simulink model "driver_model_b_upd (2)"  (R2023a)
settings: Solver=FixedStepDiscrete  StartTime=0  StopTime=700  FixedStep=0.0005  RelTol=1e-3  AbsTol=1e-6
InitFcn:
  | R2D = 180/pi;
undefined symbols (not defined in the file or in its folder): b_hat_Max, SrsLrn_BrkPedDownLim, SrsLrn_BrkPedUpLim, SrsLrn_EKF_Q1, SrsLrn_EKF_Q2, SrsLrn_ExitAccPedLim, SrsLrn_Lamda1, SrsLrn_Lamda2, SrsLrn_LongAccDownLim, SrsLrn_LongAccUpLim, SrsLrn_State1Cnt, SrsLrn_State2Cnt, SrsLrn_State5Cnt, SrsLrn_State6Cnt, SrsLrn_State7Cnt, SrsLrn_UpdBrkPedDown, SrsLrn_UpdBrkPedUp, tau_hat_Max
libraries: simulink x11, slpidlib x2, Solver_SF x1
(part 1 of 2)
settings Model: ExtModeTrigMode=oneshot  Creator=jhu  LastModifiedBy=SM-PC
settings SolverCC: AutoScaleAbsTol=off  AlgebraicLoopSolver=TrustRegion
settings DataIOCC: SaveFormat=Array  ReturnWorkspaceOutputs=off  SignalLoggingName=sigsOut
settings OptimizationCC: BlockReduction=off  BooleanDataType=off  ExpressionDepthLimit=2147483647  InitFltsAndDblsToZero=on  LifeSpan=inf
settings DebuggingCC: SaveWithParameterizedLinksMsg=none  UnderspecifiedInitializationDetection=Classic  MergeDetectMultiDrivingBlocksExec=none  SignalResolutionControl=TryResolveAllWithWarning  MultiTaskDSMMsg=warning  MultiTaskCondExecSysMsg=none  ParameterPrecisionLossMsg=none  FcnCallInpInsideContextMsg=warning  UnconnectedInputMsg=warning  UnconnectedOutputMsg=warning  UnconnectedLineMsg=warning  StateNameClashWarn=warning  SFUnexpectedBacktrackingDiag=warning  SFNoUnconditionalDefaultTransitionDiag=warning  ArithmeticOperatorsInVariantConditions=warning
settings HardwareCC: ProdBitPerPointer=32  ProdBitPerSizeT=32  ProdBitPerPtrDiffT=32  ProdLargestAtomicFloat=None  ProdIntDivRoundTo=Undefined  ProdEndianess=Unspecified  ProdWordSize=32  ProdHWDeviceType=32-bit Generic  TargetHWDeviceType=32-bit Generic  TargetUnknown=on  ProdEqTarget=off
settings ModelReferenceCC: ModelReferenceMinAlgLoopOccurrences=on  PropagateSignalLabelsOutOfModel=off
settings SFSimCC: SimUseLocalCustomCode=off  CustomCodeUndefinedFunction=UseInterfaceOnly
settings RTWCC: TemplateMakefile=grt_vc.tmf  RTWUseLocalCustomCode=off
settings CodeAppCC: StateflowObjectComments=on
settings GRTTargetCC: TargetFcnLib=ansi_tfl_tmw.mat  TargetLangStandard=C89/C90 (ANSI)  CombineOutputUpdateFcns=off  GRTInterface=on
settings ConfigComp: CovMetricSettings=dw  CovSaveCumulativeToWorkspaceVar=on  CovSaveSingleToWorkspaceVar=on  CovExternalEMLEnable=off

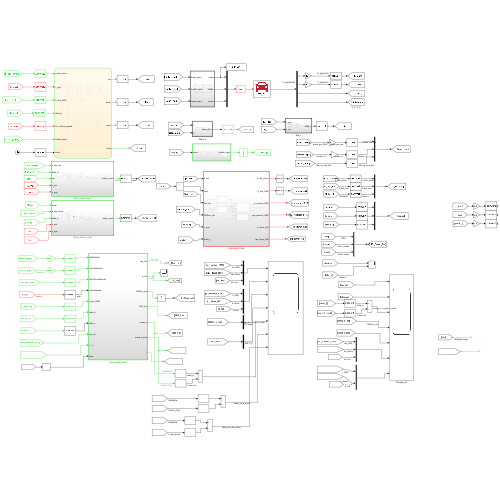
[thumbnail: Simulink's stored preview of the top-level diagram]
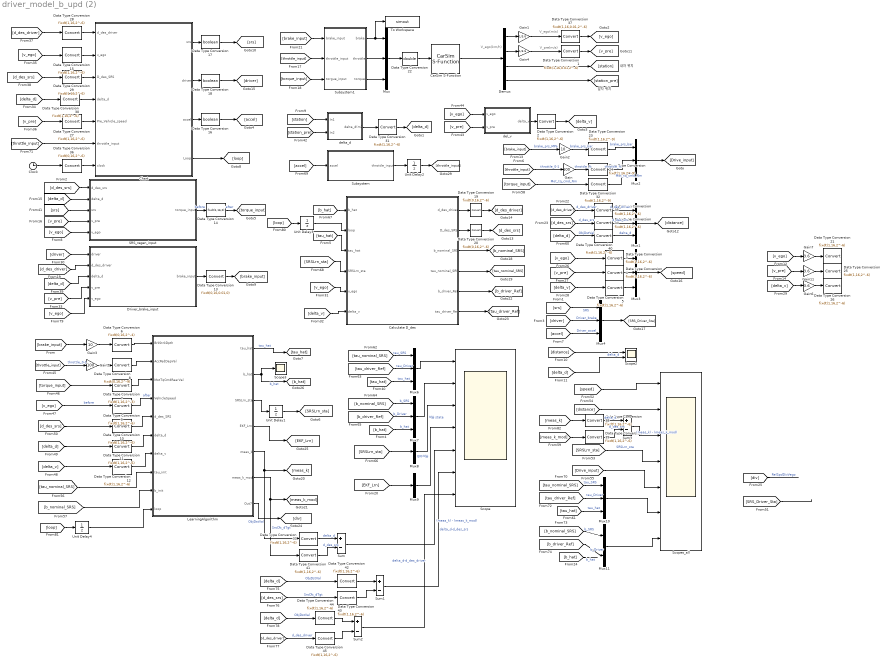
== system driver_model_b_upd (2) ==
  note: V_ego(m/s)
  note: V_pre(m/s)
  note: V_ego(km/h)
  Calculate D_des : Subsystem  TreatAsAtomicUnit=on  SystemSampleTime=0.01
      settings: MinAlgLoopOccurrences=on
  CarSim S-Function : Solver_SF/CarSim S-Function  Priority=1  SIMFILE=simfile.sim  Run_RTs=off  vs_state_ind=Run  StopMode_ind=Vehicle Model
  Chart : Stateflow chart  TreatAsAtomicUnit=on  SystemSampleTime=0.01
  Clock : Clock
  Data Type Conversion1 : DataTypeConversion  OutMin=[0]  OutMax=[300]  OutDataTypeStr=fixdt(1,16,0.01,2^-6)  RndMeth=Simplest  SaturateOnIntegerOverflow=off
  Data Type Conversion{10,29,33..35,38..45} (13 alike) : DataTypeConversion  OutDataTypeStr=fixdt(1,16,2^-6)  SaturateOnIntegerOverflow=off  RndMeth=Floor
  Data Type Conversion{2..5,9,11..12,15,21,25..27,31} (13 alike) : DataTypeConversion  OutDataTypeStr=fixdt(1,16,2^-6)  RndMeth=Simplest  SaturateOnIntegerOverflow=off
  Data Type Conversion13 : DataTypeConversion  OutDataTypeStr=fixdt(0,16,0.01,0)  SaturateOnIntegerOverflow=off  RndMeth=Floor
  Data Type Conversion14 : DataTypeConversion  OutDataTypeStr=fixdt(1,16,0)  RndMeth=Nearest  SaturateOnIntegerOverflow=off
  Data Type Conversion16 : DataTypeConversion  OutDataTypeStr=boolean  SaturateOnIntegerOverflow=off  RndMeth=Floor
  Data Type Conversion17 : DataTypeConversion  OutDataTypeStr=boolean  SaturateOnIntegerOverflow=off  RndMeth=Floor
  Data Type Conversion18 : DataTypeConversion  OutDataTypeStr=boolean  SaturateOnIntegerOverflow=off  RndMeth=Floor
  Data Type Conversion19 : DataTypeConversion  OutDataTypeStr=fixdt(0,16,2^-6)  SaturateOnIntegerOverflow=off  RndMeth=Floor
  Data Type Conversion20 : DataTypeConversion  OutDataTypeStr=fixdt(0,16,2^-6)  SaturateOnIntegerOverflow=off  RndMeth=Floor
  Data Type Conversion22 : DataTypeConversion  OutDataTypeStr=double  SaturateOnIntegerOverflow=off  RndMeth=Floor
  Data Type Conversion23 : DataTypeConversion  OutDataTypeStr=fixdt(1,16,2^-9)  SaturateOnIntegerOverflow=off  RndMeth=Floor
  Data Type Conversion24 : DataTypeConversion  OutDataTypeStr=fixdt(1,16,2^-9)  SaturateOnIntegerOverflow=off  RndMeth=Floor
  Data Type Conversion28 : DataTypeConversion  OutDataTypeStr=fixdt(1,16,2^-6)  RndMeth=Nearest  SaturateOnIntegerOverflow=off
  Data Type Conversion30 : DataTypeConversion  OutDataTypeStr=fixdt(1,16,2^-6)  RndMeth=Nearest  SaturateOnIntegerOverflow=off
  Data Type Conversion32 : DataTypeConversion  OutDataTypeStr=fixdt(1,16,2^-9)  SaturateOnIntegerOverflow=off  RndMeth=Floor
  Data Type Conversion36 : DataTypeConversion  OutDataTypeStr=fixdt(0,16,2^-6)  SaturateOnIntegerOverflow=off  RndMeth=Floor
  Data Type Conversion37 : DataTypeConversion  OutDataTypeStr=fixdt(1,16,0.01,2^-6)  RndMeth=Simplest  SaturateOnIntegerOverflow=off
  Data Type Conversion6 : DataTypeConversion  OutDataTypeStr=fixdt(0,16,2^-4)  SaturateOnIntegerOverflow=off  RndMeth=Floor
  Data Type Conversion7 : DataTypeConversion  OutDataTypeStr=fixdt(1,16,2^-3)  SaturateOnIntegerOverflow=off  RndMeth=Floor
  Data Type Conversion8 : DataTypeConversion  OutDataTypeStr=fixdt(0,16,2^-9)  SaturateOnIntegerOverflow=off  RndMeth=Floor
  Demux : Demux
  Driver_brake_input : Subsystem  TreatAsAtomicUnit=on  SystemSampleTime=0.01
  Gain : Gain  Gain=100
  Gain1 : Gain  Gain=1/3.6
  Gain11 : Gain  Gain=3.6
  Gain2 : Gain  Gain=10
  Gain3 : Gain  Gain=10
  Gain4 : Gain  Gain=1/3.6
  Gain5 : Gain  Gain=100
  Gain6 : Gain  Gain=3.6
  Gain7 : Gain  Gain=3.6
  LearningAlgorithm : Subsystem  TreatAsAtomicUnit=on  SystemSampleTime=0.01
  Mux{,1..4,6..7,10} (8 alike) : Mux  Inputs=3
  Mux11 : Mux  Inputs=2
  Mux8 : Mux  Inputs=1
  Mux9 : Mux  Inputs=1
  SRS_regen_input : Subsystem  TreatAsAtomicUnit=on  SystemSampleTime=0.01
  Scope : Scope  NumInputPorts=7
  Scope2 : Scope  NumInputPorts=2
  Scope3 : Scope
  Scopes_all : Scope  NumInputPorts=7
  Subsystem : Subsystem  TreatAsAtomicUnit=on  SystemSampleTime=0.01
      settings: MinAlgLoopOccurrences=on
  Subsystem1 : Subsystem  TreatAsAtomicUnit=on  SystemSampleTime=0.0005
  Sum{,1..3} (4 alike) : Sum  Inputs=+-
  To Workspace : ToWorkspace  VariableName=simout  SaveFormat=Timeseries  SampleTime=-1
  Unit Delay1 : UnitDelay  SampleTime=0.01  HasFrameUpgradeWarning=on
  Unit Delay2 : UnitDelay  SampleTime=0.01  HasFrameUpgradeWarning=on
  Unit Delay3 : UnitDelay  InitialCondition=1  SampleTime=0.01  HasFrameUpgradeWarning=on
  Unit Delay4 : UnitDelay  InitialCondition=1  SampleTime=0.01  HasFrameUpgradeWarning=on
  del_v : Subsystem  TreatAsAtomicUnit=on  SystemSampleTime=0.01
  delta_d : Subsystem  TreatAsAtomicUnit=on  SystemSampleTime=0.01
  wires:
  Gain1/1 -> Data Type Conversion37/1
  Mux1/1 -> [distance]
  Mux2/1 -> [Drive_input]
  [brake_input] -> Gain2/1  "brake_prs_MPa"
  [d_des_driver] -> Data Type Conversion35/1  "d_des_driver"
  [d_des_srs] -> Data Type Conversion34/1  "d_des_srs"
  [delta_d] -> Data Type Conversion30/1
  [v_pre] -> Data Type Conversion27/1
  [d_des_driver] -> Data Type Conversion28/1
  [d_des_srs] -> Data Type Conversion29/1
  Chart/1(srs) -> Data Type Conversion17/1
  Chart/2(driver) -> Data Type Conversion18/1
  [driver] -> Mux4/2  "Driver_brake"
  [srs] -> Mux4/1  "SRS"
  Mux4/1 -> [SRS_Driver_Sta]
  Chart/3(accel) -> Data Type Conversion16/1
  [throttle_input] -> Gain/1  "throttle_0-1"
  [accel] -> Mux4/3  "Driver_accel"
  Mux3/1 -> [speed]
  [d_des_driver] -> Driver_brake_input/2(d_des_driver)
  [delta_d] -> Driver_brake_input/3(delta_d)
  Driver_brake_input/1(brake_input) -> Data Type Conversion13/1
  [d_des_srs] -> SRS_regen_input/1(d_des_srs)
  [delta_d] -> SRS_regen_input/2(delta_d)
  [driver] -> Driver_brake_input/1(driver)
  [srs] -> SRS_regen_input/3(srs)
  SRS_regen_input/1(torque_input) -> Data Type Conversion14/1  "before"
  [v_pre] -> SRS_regen_input/4(v_pre)
  [v_pre] -> Driver_brake_input/4(v_pre)
  Gain4/1 -> Data Type Conversion1/1
  Demux/2 -> Gain4/1
  Gain/1 -> Data Type Conversion24/1  "throttle_%"
  Gain2/1 -> Data Type Conversion23/1  "brake_prs_bar"
  [brake_input] -> Gain3/1
  Gain3/1 -> Data Type Conversion6/1
  [throttle_input] -> Gain5/1  "throttle_0-1"
  Gain5/1 -> Data Type Conversion8/1
  [torque_input] -> Data Type Conversion7/1
  [v_ego] -> Data Type Conversion9/1  "before"
  [delta_d] -> Data Type Conversion11/1
  [d_des_srs] -> Data Type Conversion10/1
  [v_ego] -> Data Type Conversion3/1
  [v_pre] -> Data Type Conversion4/1
  [delta_v] -> Data Type Conversion5/1
  [SRS_Driver_Sta] -> ?
  [SRSLrn_sta] -> Scopes_all/4  "SRSLrn_sta"
  [speed] -> Scopes_all/1
  [distance] -> Scopes_all/2
  [Drive_input] -> Scopes_all/5
  [tau_nominal_SRS] -> LearningAlgorithm/8(tau_init)
  LearningAlgorithm/1(tau_hat) -> [tau_hat]  "tau_hat"
  LearningAlgorithm/2(b_hat) -> [b_hat], Scope3/1  "b_hat"
  Mux6/1 -> Scope/1
  Mux7/1 -> Scope/2
  [tau_nominal_SRS] -> Mux6/1  "tau_SRS"
  [tau_driver_Ref] -> Mux6/2  "tau_Driver"
  [b_nominal_SRS] -> Mux7/1  "b_SRS"
  [b_driver_Ref] -> Mux7/2  "b_Driver"
  Clock/1 -> Data Type Conversion36/1
  [b_nominal_SRS] -> LearningAlgorithm/9(b_init)
  LearningAlgorithm/3(SRSLrn_sta) -> Unit Delay1/1
  Unit Delay1/1 -> [SRSLrn_sta]
  LearningAlgorithm/4(EKF_Lrn) -> [EKF_Lrn]
  [EKF_Lrn] -> Mux9/1
  [SRSLrn_sta] -> Mux8/1
  Mux8/1 -> Scope/3  "학습 state"
  Mux9/1 -> Scope/4  "EKF학습"
  [b_hat] -> Mux7/3  "b_hat"
  [tau_hat] -> Mux6/3  "tau_hat"
  [accel] -> Subsystem/1(accel)
  Calculate D_des/3(b_nominal_SRS) -> [b_nominal_SRS]
  [tau_hat] -> Calculate D_des/3(tau_hat)
  Calculate D_des/6(tau_driver_Ref) -> [tau_driver_Ref]
  Calculate D_des/4(tau_nominal_SRS) -> [tau_nominal_SRS]
  Calculate D_des/1(d_des_driver) -> Data Type Conversion19/1
  Calculate D_des/5(b_driver_Ref) -> [b_driver_Ref]
  [SRSLrn_sta] -> Calculate D_des/4(SRSLrn_sta)
  Calculate D_des/2(D_des_SRS) -> Data Type Conversion20/1
  [v_ego] -> Calculate D_des/5(v_ego)
  [delta_v] -> Calculate D_des/6(delta_v)
  [b_hat] -> Calculate D_des/1(b_hat)
  CarSim S-Function/1 -> Demux/1
  Data Type Conversion37/1 -> [v_ego]
  Data Type Conversion1/1 -> [v_pre]
  Data Type Conversion2/1 -> [delta_v]
  Data Type Conversion3/1 -> Mux3/1
  Data Type Conversion4/1 -> Mux3/2
  Data Type Conversion5/1 -> Mux3/3
  Data Type Conversion6/1 -> LearningAlgorithm/1(BrkStrkDpth)
  Data Type Conversion8/1 -> LearningAlgorithm/2(AccPedDepVal)
  Data Type Conversion7/1 -> LearningAlgorithm/3(MotTqCmdRearVal)
  Data Type Conversion9/1 -> LearningAlgorithm/4(VehicleSpeed)  "after"
  Data Type Conversion10/1 -> LearningAlgorithm/5(d_des_SRS)
  Data Type Conversion11/1 -> LearningAlgorithm/6(delta_d)
  Data Type Conversion12/1 -> LearningAlgorithm/7(delta_v)
  Mux/1 -> Data Type Conversion22/1
  Data Type Conversion14/1 -> [torque_input]  "after"
  Data Type Conversion16/1 -> [accel]
  Data Type Conversion17/1 -> [srs]
  Data Type Conversion18/1 -> [driver]
  Subsystem/1(throttle_input) -> Unit Delay2/1
  Data Type Conversion19/1 -> [d_des_driver]
  Data Type Conversion20/1 -> [d_des_srs]
  Data Type Conversion22/1 -> CarSim S-Function/1
  Data Type Conversion23/1 -> Mux2/1  "brake_prs_bar"
  Data Type Conversion24/1 -> Mux2/2  "throttle_%"
  Data Type Conversion15/1 -> Chart/2(v_ego)
  Data Type Conversion28/1 -> Chart/1(d_des_driver)
  Data Type Conversion29/1 -> Chart/3(D_des_SRS)
  Data Type Conversion30/1 -> Chart/4(delta_d)
  Data Type Conversion27/1 -> Chart/5(Pre_Vehicle_speed)
  [throttle_input] -> Chart/6(throttle_input)
  Data Type Conversion34/1 -> Mux1/2  "d_des_srs"
  Data Type Conversion35/1 -> Mux1/1  "d_des_driver"
  Data Type Conversion13/1 -> [brake_input]
  Data Type Conversion36/1 -> Chart/7(clock)
  Demux/1 -> Gain1/1
  [v_ego] -> SRS_regen_input/5(v_ego)
  [v_ego] -> Data Type Conversion15/1
  [distance] -> Scope2/1
  [delta_d] -> Scope2/2  "delta_d"
  Demux/3 -> [station]
  Demux/4 -> [station_pre]
  Data Type Conversion31/1 -> [delta_d]
  [v_ego] -> del_v/1(v_ego)
  [v_pre] -> del_v/2(v_pre)
  del_v/1(delta_v) -> Data Type Conversion2/1
  [station] -> delta_d/1(In1)
  [station_pre] -> delta_d/2(In2)
  delta_d/1(delta_d(m)) -> Data Type Conversion31/1
  [brake_input] -> Subsystem1/1(brake_input)
  [throttle_input] -> Subsystem1/2(throttle_input)
  [torque_input] -> Subsystem1/3(torgue_input)
  Subsystem1/1(brake) -> To Workspace/1, Mux/1
  Subsystem1/2(throttle) -> Mux/2
  Subsystem1/3(torque) -> Mux/3
  [delta_v] -> Data Type Conversion12/1
  Gain6/1 -> Data Type Conversion26/1
  [delta_v] -> Gain6/1
  [v_pre] -> Gain11/1
  Gain11/1 -> Data Type Conversion25/1
  [v_ego] -> Gain7/1
  Gain7/1 -> Data Type Conversion21/1
  [torque_input] -> Data Type Conversion32/1  "Mot_tq_cmd_Nm"
  Data Type Conversion32/1 -> Mux2/3  "Mot_tq_cmd_Nm"
  [delta_d] -> Data Type Conversion40/1  "ObjDstVal"
  Data Type Conversion40/1 -> Mux1/3  "delta_d"
  Mux10/1 -> Scopes_all/6
  [b_driver_Ref] -> Mux11/2  "b_Driver"
  [b_nominal_SRS] -> Mux11/1  "b_SRS"
  Mux11/1 -> Scopes_all/7
  [tau_driver_Ref] -> Mux10/2  "tau_Driver"
  [tau_nominal_SRS] -> Mux10/1  "tau_SRS"
  [tau_hat] -> Mux10/3  "tau_hat"
  [b_hat] -> ?  "b_hat"
  Sum/1 -> Scope/5  "(meas_k) - (meas_k_mod)"
  Data Type Conversion41/1 -> Sum/2  "d_des_srs"
  LearningAlgorithm/5(meas_k) -> Data Type Conversion33/1, [meas_k]  "ObjDstVal"
  Data Type Conversion33/1 -> Sum/1  "delta_d"
  LearningAlgorithm/6(meas_k_mod) -> Data Type Conversion41/1, [meas_k_mod]  "SrsCfc_dTgt"
  Data Type Conversion43/1 -> Sum1/2
  Data Type Conversion42/1 -> Sum1/1
  Sum1/1 -> Scope/6  "delta_d-d_des_srs"
  [delta_d] -> Data Type Conversion42/1  "ObjDstVal"
  [d_des_srs] -> Data Type Conversion43/1  "SrsCfc_dTgt"
  Chart/4(Loop) -> [loop]
  Data Type Conversion44/1 -> Sum2/1
  Data Type Conversion45/1 -> Sum2/2
  [delta_d] -> Data Type Conversion44/1  "ObjDstVal"
  [d_des_driver] -> Data Type Conversion45/1  "d_des_driver"
  Sum2/1 -> Scope/7  "delta_d-d_des_driver"
  [v_ego] -> Driver_brake_input/5(v_ego)
  [loop] -> Unit Delay3/1
  Unit Delay3/1 -> Calculate D_des/2(loop)
  [loop] -> Unit Delay4/1
  Unit Delay4/1 -> LearningAlgorithm/10(loop)
  Unit Delay2/1 -> [throttle_input]
  LearningAlgorithm/7(Out7) -> [div]
  [div] -> ?  "RelSpdDivVego"
  Data Type Conversion39/1 -> Sum3/2  "d_des_srs"
  Data Type Conversion38/1 -> Sum3/1  "delta_d"
  [meas_k] -> Data Type Conversion38/1
  [meas_k_mod] -> Data Type Conversion39/1
  Sum3/1 -> Scopes_all/3  "(meas_k) - (meas_k_mod)"

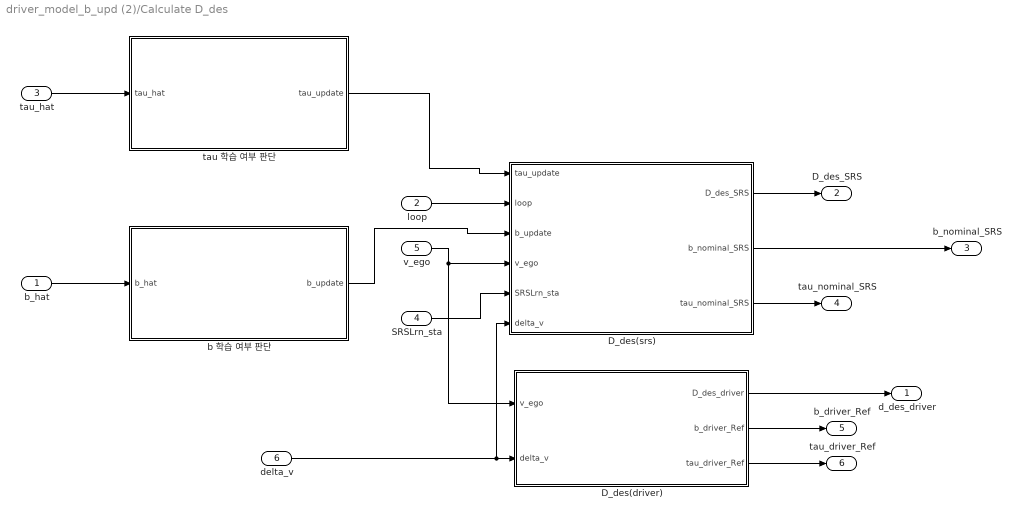
== system driver_model_b_upd (2)/Calculate D_des ==
  b_hat : Inport
  loop : Inport  Port=2
  tau_hat : Inport  Port=3
  SRSLrn_sta : Inport  Port=4
  v_ego : Inport  Port=5
  delta_v : Inport  Port=6
  D_des(driver) : Subsystem
  D_des(srs) : Subsystem
  b 학습 여부 판단 : Subsystem
  tau 학습 여부 판단 : Subsystem
  d_des_driver : Outport
  D_des_SRS : Outport  Port=2
  b_nominal_SRS : Outport  Port=3
  tau_nominal_SRS : Outport  Port=4
  b_driver_Ref : Outport  Port=5
  tau_driver_Ref : Outport  Port=6
  wires:
  v_ego/1 -> D_des(driver)/1(v_ego), D_des(srs)/4(v_ego)
  delta_v/1 -> D_des(driver)/2(delta_v), D_des(srs)/6(delta_v)
  D_des(srs)/1(D_des_SRS) -> D_des_SRS/1
  D_des(driver)/1(D_des_driver) -> d_des_driver/1
  D_des(srs)/2(b_nominal_SRS) -> b_nominal_SRS/1
  D_des(srs)/3(tau_nominal_SRS) -> tau_nominal_SRS/1
  D_des(driver)/2(b_driver_Ref) -> b_driver_Ref/1
  D_des(driver)/3(tau_driver_Ref) -> tau_driver_Ref/1
  SRSLrn_sta/1 -> D_des(srs)/5(SRSLrn_sta)
  b_hat/1 -> b 학습 여부 판단/1(b_hat)
  b 학습 여부 판단/1(b_update) -> D_des(srs)/3(b_update)
  tau_hat/1 -> tau 학습 여부 판단/1(tau_hat)
  tau 학습 여부 판단/1(tau_update) -> D_des(srs)/1(tau_update)
  loop/1 -> D_des(srs)/2(loop)

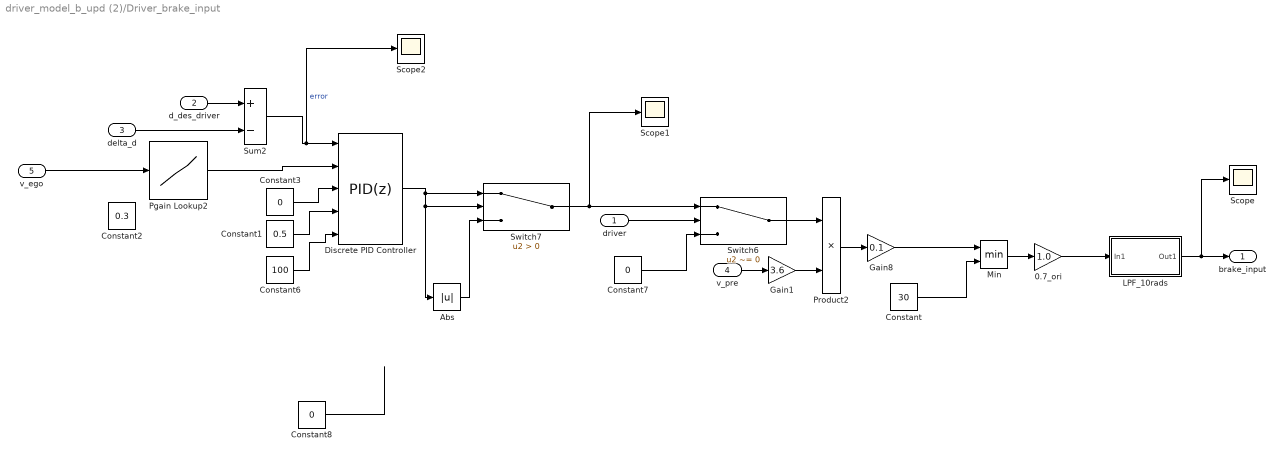
== system driver_model_b_upd (2)/Driver_brake_input ==
  driver : Inport
  d_des_driver : Inport  Port=2
  delta_d : Inport  Port=3
  v_pre : Inport  Port=4
  v_ego : Inport  Port=5
  0.7_ori : Gain  Gain=1.0
  Abs : Abs  SaturateOnIntegerOverflow=off
  Constant : Constant  Value=30
  Constant1 : Constant  Value=0.5
  Constant2 : Constant  Value=0.3
  Constant3 : Constant  Value=0
  Constant6 : Constant  Value=100
  Constant7 : Constant  Value=0
  Constant8 : Constant  Value=0
  Discrete PID Controller : slpidlib/PID Controller  Controller=PID  Form=Parallel  TimeDomain=Discrete-time  UseExternalTs=off  SampleTime=0.01  IntegratorMethod=Forward Euler  FilterMethod=Forward Euler  ControllerParametersSource=external  P=1  I=1  UseKiTs=off  D=0  N=100  UseFilter=on  TunerSelectOption=Transfer Function Based (PID Tuner App)  InitialConditionSource=internal  InitialConditionForIntegrator=0  InitialConditionForFilter=0  DifferentiatorICPrevScaledInput=0  ExternalReset=none  TrackingMode=off  Kt=1  LimitOutput=off  SatLimitsSource=internal  UpperSaturationLimit=inf  LowerSaturationLimit=-inf  LinearizeAsGain=off  AntiWindupMode=none  Kb=1  LimitIntegrator=off  UpperIntegratorSaturationLimit=inf  LowerIntegratorSaturationLimit=-inf  POutMin=[]  POutMax=[]  IOutMin=[]  IOutMax=[]  DOutMin=[]  DOutMax=[]  NOutMin=[]  NOutMax=[]  SumOutMin=[]  SumOutMax=[]  SaturationOutMin=[]  SaturationOutMax=[]  PParamMin=[]  PParamMax=[]  IParamMin=[]  IParamMax=[]  DParamMin=[]  DParamMax=[]  NParamMin=[]  NParamMax=[]  KbParamMin=[]  KbParamMax=[]  KtParamMin=[]  KtParamMax=[]  KbOutMin=[]  KbOutMax=[]  KtOutMin=[]  KtOutMax=[]  IntegratorOutMin=[]  IntegratorOutMax=[]  FilterOutMin=[]  FilterOutMax=[]  SumI1OutMin=[]  SumI1OutMax=[]  SumI2OutMin=[]  SumI2OutMax=[]  SumI3OutMin=[]  SumI3OutMax=[]  SumI4OutMin=[]  SumI4OutMax=[]  SumDOutMin=[]  SumDOutMax=[]  DifferentiatorOutMin=[]  DifferentiatorOutMax=[]  FilterDiffOutCoefMin=[]  FilterDiffOutCoefMax=[]  ReciprocalOutMin=[]  ReciprocalOutMax=[]  SumDenOutMin=[]  SumDenOutMax=[]  SumNumOutMin=[]  SumNumOutMax=[]  DivideOutMin=[]  DivideOutMax=[]  UdiffTsProdOutMin=[]  UdiffTsProdOutMax=[]  NTsProdOutMin=[]  NTsProdOutMax=[]  UintegralTsProdOutMin=[]  UintegralTsProdOutMax=[]  UngainTsProdOutMin=[]  UngainTsProdOutMax=[]  ClampingZeroOutDataTypeStr=Inherit: Inherit via back propagation  ClampingZeroOutMin=[]  ClampingZeroOutMax=[]  FilterDenConstantOutDataTypeStr=Inherit: Inherit via back propagation  FilterDenConstantOutMin=[]  FilterDenConstantOutMax=[]  PCopyOutDataTypeStr=Inherit: Inherit via back propagation  PCopyOutMin=[]  PCopyOutMax=[]  NCopyOutDataTypeStr=Inherit: Inherit via back propagation  NCopyOutMin=[]  NCopyOutMax=[]  IntegratorContinuousStateAttributes=''  IntegratorStateMustResolveToSignalObject=off  IntegratorRTWStateStorageClass=Auto  FilterContinuousStateAttributes=''  FilterStateMustResolveToSignalObject=off  FilterRTWStateStorageClass=Auto  ParallelPVariant=ExternalParameters  IdealPVariant=Disabled  IVariant=ExternalParameters  DVariant=ExternalParameters  IntegratorVariant=Discrete  SatVariant=Disabled  AWVariant=Passthrough  PCopyVariant=Disabled  TRVariant=Disabled  FdbkBlocksVariant=Forward  IdealPFdbkVariant=Disabled  SatFdbkVariant=Disabled  DerivativeFilterVariant=ForwardEulerFilter  NVariant=ExternalParameters  NCopyVariant=Disabled  FilterICVariant=InternalICsFilter  IntegratorICVariant=InternalICs  ExternalResetVariant=Disabled  TRSumVariant=Passthrough  SumFdbkVariant=Disabled  SumVariant=Sum_PID  TsampFilterVariant=InternalTs  TsampNgainVariant=Passthrough  TsampIntegralVariant=Disabled_SignalSpec  ExternalSaturationOutDataTypeStr=Inherit: Same as second input
  Gain1 : Gain  Gain=3.6
  Gain8 : Gain  Gain=0.1
  LPF_10rads : Subsystem
  Min : MinMax  Inputs=2
  Pgain Lookup2 : Lookup_n-D  NumberOfTableDimensions=1  BreakpointsForDimension1=[0 2 4 6 8 10 12 14 16 18 20]  Table=[0.2 0.2 0.2 0.2 0.2 0.2 0.2 0.2 0.3 0.3 0.3 ]  ExtrapMethod=Clip  UseLastTableValue=on  InternalRulePriority=Speed  RndMeth=Simplest
  Product2 : Product  SaturateOnIntegerOverflow=on  OutDataTypeStr=Inherit: Same as first input
  Scope : Scope
  Scope1 : Scope
  Scope2 : Scope
  Sum2 : Sum  Inputs=+-
  Switch6 : Switch  Criteria=u2 ~= 0  SaturateOnIntegerOverflow=off  InputSameDT=off
  Switch7 : Switch  Criteria=u2 > Threshold  SaturateOnIntegerOverflow=off  InputSameDT=off
  brake_input : Outport
  wires:
  Constant6/1 -> Discrete PID Controller/5
  Discrete PID Controller/1 -> Abs/1, Switch7/2, Switch7/1
  Sum2/1 -> Scope2/1, Discrete PID Controller/1  "error"
  Product2/1 -> Gain8/1
  Constant7/1 -> Switch6/3
  d_des_driver/1 -> Sum2/1
  Constant8/1 -> ?
  Switch7/1 -> Scope1/1, Switch6/1
  Switch6/1 -> Product2/1
  driver/1 -> Switch6/2
  v_pre/1 -> Gain1/1
  Gain1/1 -> Product2/2
  Constant1/1 -> Discrete PID Controller/4
  Min/1 -> 0.7_ori/1
  LPF_10rads/1(Out1) -> Scope/1, brake_input/1
  Constant/1 -> Min/2
  0.7_ori/1 -> LPF_10rads/1(In1)
  Constant3/1 -> Discrete PID Controller/3
  Gain8/1 -> Min/1
  delta_d/1 -> Sum2/2
  Abs/1 -> Switch7/3
  v_ego/1 -> Pgain Lookup2/1
  Pgain Lookup2/1 -> Discrete PID Controller/2

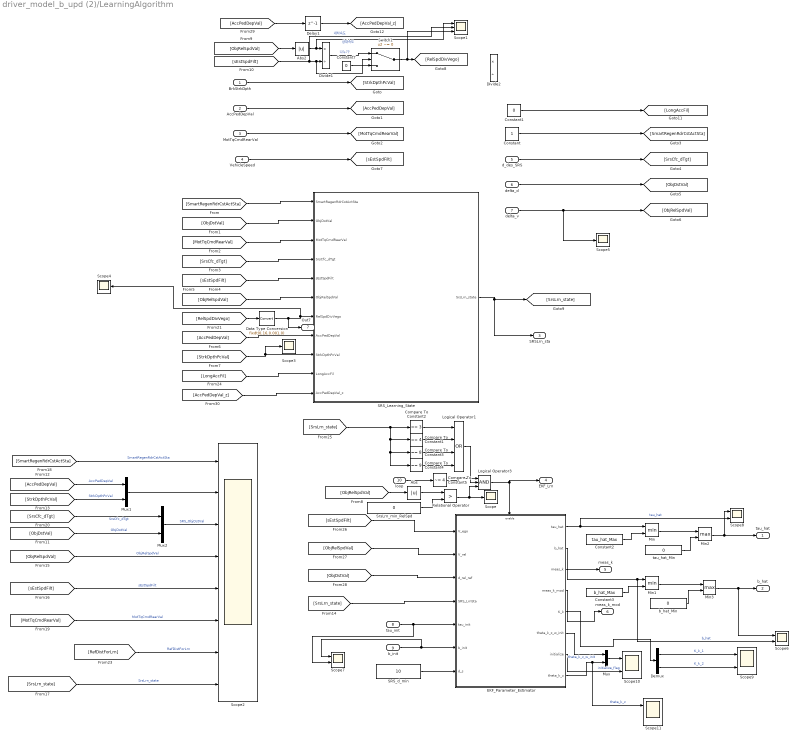
== system driver_model_b_upd (2)/LearningAlgorithm ==
  BrkStrkDpth : Inport
  AccPedDepVal : Inport  Port=2
  MotTqCmdRearVal : Inport  Port=3
  VehicleSpeed : Inport  Port=4
  d_des_SRS : Inport  Port=5
  delta_d : Inport  Port=6
  delta_v : Inport  Port=7
  tau_init : Inport  Port=8
  b_init : Inport  Port=9
  loop : Inport  Port=10
  Abs : Abs  SaturateOnIntegerOverflow=off
  Abs2 : Abs  SaturateOnIntegerOverflow=off
  Compare To Constant1 : simulink/Logic and Bit Operations/Compare To Constant  relop===  const=4  OutDataTypeStr=boolean
  Compare To Constant2 : simulink/Logic and Bit Operations/Compare To Constant  relop===  const=3  OutDataTypeStr=boolean
  Compare To Constant3 : simulink/Logic and Bit Operations/Compare To Constant  relop===  const=8  OutDataTypeStr=boolean
  Compare To Constant4 : simulink/Logic and Bit Operations/Compare To Constant  relop===  const=9  OutDataTypeStr=boolean
  Compare To Constant5 : simulink/Logic and Bit Operations/Compare To Constant  relop=~=  const=4  OutDataTypeStr=boolean
  Constant : Constant  OutDataTypeStr=boolean
  Constant1 : Constant  Value=0  OutDataTypeStr=fixdt(1,16,2^-11)
  Constant2 : Constant  Value=tau_hat_Max
  Constant3 : Constant  Value=b_hat_Max
  Constant7 : Constant  Value=0  OutDataTypeStr=fixdt(1,16)
  Data Type Conversion : DataTypeConversion  OutDataTypeStr=fixdt(0,16,0.001,0)  RndMeth=Simplest  SaturateOnIntegerOverflow=off
  Delay1 : Delay  DelayLength=1
  Demux : Demux  Outputs=2
  Divide1 : Product  Inputs=*/  OutDataTypeStr=fixdt(1,16,0.01,2^-4)  RndMeth=Nearest
  Divide2 : Product  Inputs=*/  OutDataTypeStr=fixdt(1,16,2^-6)  RndMeth=Nearest
  EKF_Parameter_Estimator : Subsystem
  Logical Operator1 : Logic  Operator=OR  Inputs=4  AllPortsSameDT=off  OutDataTypeStr=boolean
  Logical Operator3 : Logic  Inputs=3  AllPortsSameDT=off  OutDataTypeStr=boolean
  Min : MinMax  Inputs=2
  Min1 : MinMax  Inputs=2
  Min2 : MinMax  Function=max  Inputs=2
  Min3 : MinMax  Function=max  Inputs=2
  Mux : Mux  Inputs=2
  Mux1 : Mux  Inputs=2
  Mux2 : Mux  Inputs=2
  Relational Operator : RelationalOperator  Operator=>  OutDataTypeStr=boolean  InputSameDT=off
  SRS_Learning_State : Stateflow chart  TreatAsAtomicUnit=on  SystemSampleTime=0.01
  SRS_d_min : Constant  Value=10
  Scope{,3..5} (4 alike) : Scope
  Scope1 : Scope  NumInputPorts=3
  Scope{6..11} (6 alike) : Scope  NumInputPorts=2
  Scope2 : Scope  NumInputPorts=8
  SrsLrn_min_RelSpd : Constant  Value=0
  Switch1 : Switch  Criteria=u2 ~= 0  SaturateOnIntegerOverflow=off  InputSameDT=off
  b_hat_Min : Constant  Value=0
  tau_hat_Min : Constant  Value=0
  tau_hat : Outport
  b_hat : Outport  Port=2
  SRSLrn_sta : Outport  Port=3
  EKF_Lrn : Outport  Port=4
  meas_k : Outport  Port=5
  meas_k_mod : Outport  Port=6
  Out7 : Outport  Port=7
  wires:
  [ObjDstVal] -> EKF_Parameter_Estimator/3(d_rel_ref)
  delta_v/1 -> Scope5/1, [ObjRelSpdVal]
  [ObjDstVal] -> SRS_Learning_State/2(ObjDstVal)
  [SrsCfc_dTgt] -> SRS_Learning_State/4(SrsCfc_dTgt)
  [AccPedDepVal] -> SRS_Learning_State/8(AccPedDepVal)
  [StrkDpthPcVal] -> Scope3/1, SRS_Learning_State/9(StrkDpthPcVal)
  d_des_SRS/1 -> [SrsCfc_dTgt]
  BrkStrkDpth/1 -> [StrkDpthPcVal]
  [SmartRegenRdrCstActSta] -> SRS_Learning_State/1(SmartRegenRdrCstActSta)
  [MotTqCmdRearVal] -> SRS_Learning_State/3(MotTqCmdRearVal)
  [sEstSpdFilt] -> SRS_Learning_State/5(sEstSpdFilt)
  VehicleSpeed/1 -> [sEstSpdFilt]
  MotTqCmdRearVal/1 -> [MotTqCmdRearVal]
  [ObjRelSpdVal] -> SRS_Learning_State/6(ObjRelSpdVal)
  AccPedDepVal/1 -> [AccPedDepVal]
  [ObjRelSpdVal] -> EKF_Parameter_Estimator/2(V_rel)
  delta_d/1 -> [ObjDstVal]
  [SrsLrn_state] -> Scope2/8  "SrsLrn_state"
  [MotTqCmdRearVal] -> Scope2/6  "MotTqCmdRearVal"
  [RefDistForLrn] -> Scope2/7  "RefDistForLrn"
  [ObjDstVal] -> Mux2/2  "ObjDstVal"
  Constant1/1 -> [LongAccFil]
  [LongAccFil] -> SRS_Learning_State/10(LongAccFil)
  Mux2/1 -> Scope2/3  "SRS_ObjDstVal"
  [SmartRegenRdrCstActSta] -> Scope2/1  "SmartRegenRdrCstActSta"
  [SrsLrn_state] -> EKF_Parameter_Estimator/4(SRS_LrnSta)
  Mux1/1 -> Scope2/2
  [sEstSpdFilt] -> Scope2/5  "sEstSpdFilt"
  [AccPedDepVal] -> Mux1/1  "AccPedDepVal"
  SRS_Learning_State/1(SrsLrn_state) -> SRSLrn_sta/1, [SrsLrn_state]
  [StrkDpthPcVal] -> Mux1/2  "StrkDpthPcVal"
  [SrsCfc_dTgt] -> Mux2/1  "SrsCfc_dTgt"
  [ObjRelSpdVal] -> Scope2/4  "ObjRelSpdVel"
  EKF_Parameter_Estimator/1(tau_hat) -> Scope8/2, Min/1  "tau_hat"
  EKF_Parameter_Estimator/2(b_hat) -> Scope6/2, Min1/1  "b_hat"
  tau_init/1 -> Scope7/2, EKF_Parameter_Estimator/5(tau_init)
  b_init/1 -> Scope7/1, EKF_Parameter_Estimator/6(b_init)
  EKF_Parameter_Estimator/3(meas_k) -> meas_k/1
  EKF_Parameter_Estimator/4(meas_k_mod) -> meas_k_mod/1
  Logical Operator3/1 -> EKF_Lrn/1, EKF_Parameter_Estimator/Enable
  [sEstSpdFilt] -> Scope1/2, Switch1/2, Divide1/2  "내차속도"
  Abs2/1 -> Scope1/1, Divide1/1  "상대속도"
  [ObjRelSpdVal] -> Abs2/1
  Delay1/1 -> [AccPedDepVal_z]
  [AccPedDepVal] -> Delay1/1
  [AccPedDepVal_z] -> SRS_Learning_State/11(AccPedDepVal_z)
  [RelSpdDivVego] -> Data Type Conversion/1
  Constant2/1 -> Min/2
  Constant3/1 -> Min1/2
  SRS_d_min/1 -> EKF_Parameter_Estimator/7(d_s)
  [SrsLrn_state] -> Compare To Constant2/1, Compare To Constant4/1, Compare To Constant3/1, Compare To Constant1/1
  Logical Operator1/1 -> Logical Operator3/2
  [ObjRelSpdVal] -> Abs/1
  Abs/1 -> Relational Operator/1
  Relational Operator/1 -> Scope/1, Logical Operator3/3
  SrsLrn_min_RelSpd/1 -> Relational Operator/2
  Compare To Constant1/1 -> Logical Operator1/2
  Compare To Constant3/1 -> Logical Operator1/3
  Compare To Constant4/1 -> Logical Operator1/4
  Compare To Constant2/1 -> Logical Operator1/1
  Data Type Conversion/1 -> Out7/1, SRS_Learning_State/7(RelSpdDivVego), Scope4/1
  Min/1 -> Min2/1
  Min1/1 -> Min3/1
  tau_hat_Min/1 -> Min2/2
  Min2/1 -> Scope8/1, tau_hat/1
  b_hat_Min/1 -> Min3/2
  Min3/1 -> Scope6/1, b_hat/1
  [sEstSpdFilt] -> EKF_Parameter_Estimator/1(V_ego)
  Switch1/1 -> Scope1/3, [RelSpdDivVego]
  Divide1/1 -> Switch1/1  "나누기'"
  Constant7/1 -> Switch1/3
  Constant/1 -> [SmartRegenRdrCstActSta]
  EKF_Parameter_Estimator/5(K_k) -> Demux/1
  Demux/1 -> Scope9/1  "K_k_1"
  Demux/2 -> Scope9/2  "K_k_2"
  EKF_Parameter_Estimator/6(theta_k_z_w_init) -> Mux/1  "theta_k_z_w_init"
  EKF_Parameter_Estimator/7(initialize) -> Scope10/2  "initialize_flag"
  EKF_Parameter_Estimator/8(theta_k_z) -> Scope11/1, Mux/2  "theta_k_z"
  Mux/1 -> Scope10/1
  loop/1 -> Compare To Constant5/1
  Compare To Constant5/1 -> Logical Operator3/1

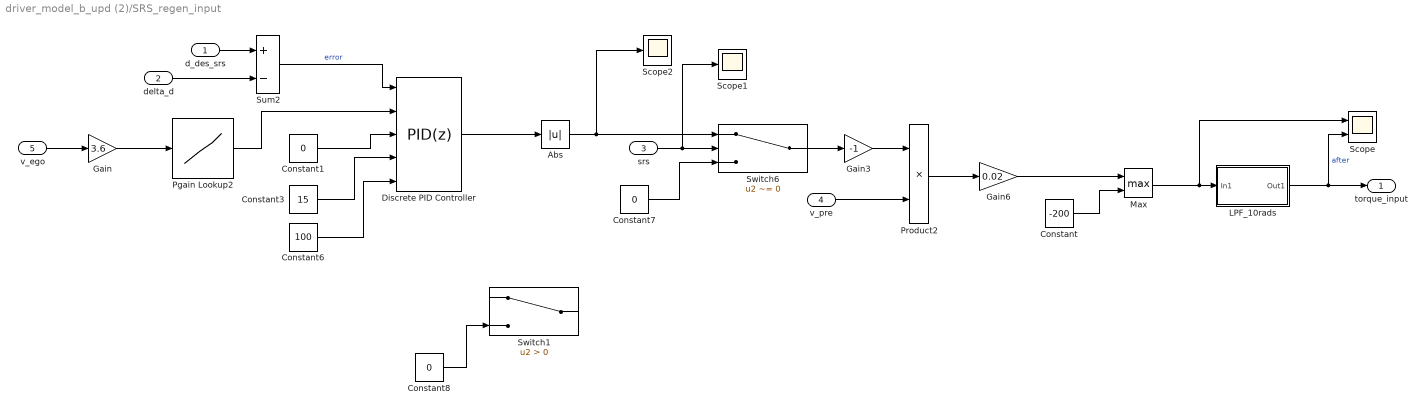
== system driver_model_b_upd (2)/SRS_regen_input ==
  d_des_srs : Inport
  delta_d : Inport  Port=2
  srs : Inport  Port=3
  v_pre : Inport  Port=4
  v_ego : Inport  Port=5
  Abs : Abs  SaturateOnIntegerOverflow=off
  Constant : Constant  Value=-200
  Constant1 : Constant  Value=0
  Constant3 : Constant  Value=15
  Constant6 : Constant  Value=100
  Constant7 : Constant  Value=0
  Constant8 : Constant  Value=0
  Discrete PID Controller : slpidlib/PID Controller  Controller=PID  Form=Parallel  TimeDomain=Discrete-time  UseExternalTs=off  SampleTime=0.01  IntegratorMethod=Forward Euler  FilterMethod=Forward Euler  ControllerParametersSource=external  P=1  I=1  UseKiTs=off  D=0  N=100  UseFilter=on  TunerSelectOption=Transfer Function Based (PID Tuner App)  InitialConditionSource=internal  InitialConditionForIntegrator=0  InitialConditionForFilter=0  DifferentiatorICPrevScaledInput=0  ExternalReset=none  TrackingMode=off  Kt=1  LimitOutput=off  SatLimitsSource=internal  UpperSaturationLimit=inf  LowerSaturationLimit=-inf  LinearizeAsGain=off  AntiWindupMode=none  Kb=1  LimitIntegrator=off  UpperIntegratorSaturationLimit=inf  LowerIntegratorSaturationLimit=-inf  POutMin=[]  POutMax=[]  IOutMin=[]  IOutMax=[]  DOutMin=[]  DOutMax=[]  NOutMin=[]  NOutMax=[]  SumOutMin=[]  SumOutMax=[]  SaturationOutMin=[]  SaturationOutMax=[]  PParamMin=[]  PParamMax=[]  IParamMin=[]  IParamMax=[]  DParamMin=[]  DParamMax=[]  NParamMin=[]  NParamMax=[]  KbParamMin=[]  KbParamMax=[]  KtParamMin=[]  KtParamMax=[]  KbOutMin=[]  KbOutMax=[]  KtOutMin=[]  KtOutMax=[]  IntegratorOutMin=[]  IntegratorOutMax=[]  FilterOutMin=[]  FilterOutMax=[]  SumI1OutMin=[]  SumI1OutMax=[]  SumI2OutMin=[]  SumI2OutMax=[]  SumI3OutMin=[]  SumI3OutMax=[]  SumI4OutMin=[]  SumI4OutMax=[]  SumDOutMin=[]  SumDOutMax=[]  DifferentiatorOutMin=[]  DifferentiatorOutMax=[]  FilterDiffOutCoefMin=[]  FilterDiffOutCoefMax=[]  ReciprocalOutMin=[]  ReciprocalOutMax=[]  SumDenOutMin=[]  SumDenOutMax=[]  SumNumOutMin=[]  SumNumOutMax=[]  DivideOutMin=[]  DivideOutMax=[]  UdiffTsProdOutMin=[]  UdiffTsProdOutMax=[]  NTsProdOutMin=[]  NTsProdOutMax=[]  UintegralTsProdOutMin=[]  UintegralTsProdOutMax=[]  UngainTsProdOutMin=[]  UngainTsProdOutMax=[]  ClampingZeroOutDataTypeStr=Inherit: Inherit via back propagation  ClampingZeroOutMin=[]  ClampingZeroOutMax=[]  FilterDenConstantOutDataTypeStr=Inherit: Inherit via back propagation  FilterDenConstantOutMin=[]  FilterDenConstantOutMax=[]  PCopyOutDataTypeStr=Inherit: Inherit via back propagation  PCopyOutMin=[]  PCopyOutMax=[]  NCopyOutDataTypeStr=Inherit: Inherit via back propagation  NCopyOutMin=[]  NCopyOutMax=[]  IntegratorContinuousStateAttributes=''  IntegratorStateMustResolveToSignalObject=off  IntegratorRTWStateStorageClass=Auto  FilterContinuousStateAttributes=''  FilterStateMustResolveToSignalObject=off  FilterRTWStateStorageClass=Auto  ParallelPVariant=ExternalParameters  IdealPVariant=Disabled  IVariant=ExternalParameters  DVariant=ExternalParameters  IntegratorVariant=Discrete  SatVariant=Disabled  AWVariant=Passthrough  PCopyVariant=Disabled  TRVariant=Disabled  FdbkBlocksVariant=Forward  IdealPFdbkVariant=Disabled  SatFdbkVariant=Disabled  DerivativeFilterVariant=ForwardEulerFilter  NVariant=ExternalParameters  NCopyVariant=Disabled  FilterICVariant=InternalICsFilter  IntegratorICVariant=InternalICs  ExternalResetVariant=Disabled  TRSumVariant=Passthrough  SumFdbkVariant=Disabled  SumVariant=Sum_PID  TsampFilterVariant=InternalTs  TsampNgainVariant=Passthrough  TsampIntegralVariant=Disabled_SignalSpec  ExternalSaturationOutDataTypeStr=Inherit: Same as second input
  Gain : Gain  Gain=3.6
  Gain3 : Gain  Gain=-1
  Gain6 : Gain  Gain=0.02
  LPF_10rads : Subsystem
  Max : MinMax  Function=max  Inputs=2
  Pgain Lookup2 : Lookup_n-D  NumberOfTableDimensions=1  BreakpointsForDimension1=[0 5 10 15 20 30 40 50 60 70 80 90 100 ]  Table=[45 45 50 50 50 50 50 50 50 55 55 55 55]  ExtrapMethod=Clip  UseLastTableValue=on  InternalRulePriority=Speed  RndMeth=Simplest
  Product2 : Product  SaturateOnIntegerOverflow=on  OutDataTypeStr=Inherit: Same as first input
  Scope : Scope  NumInputPorts=2
  Scope1 : Scope
  Scope2 : Scope
  Sum2 : Sum  Inputs=+-
  Switch1 : Switch  Criteria=u2 > Threshold  SaturateOnIntegerOverflow=off  InputSameDT=off
  Switch6 : Switch  Criteria=u2 ~= 0  SaturateOnIntegerOverflow=off  InputSameDT=off
  torque_input : Outport
  wires:
  Constant6/1 -> Discrete PID Controller/5
  Sum2/1 -> Discrete PID Controller/1  "error"
  Constant7/1 -> Switch6/3
  Constant3/1 -> Discrete PID Controller/4
  srs/1 -> Scope1/1, Switch6/2
  Constant8/1 -> Switch1/3
  Abs/1 -> Scope2/1, Switch6/1
  Product2/1 -> Gain6/1
  LPF_10rads/1(Out1) -> Scope/2, torque_input/1  "after"
  delta_d/1 -> Sum2/2
  d_des_srs/1 -> Sum2/1
  Constant1/1 -> Discrete PID Controller/3
  Gain3/1 -> Product2/1
  Switch6/1 -> Gain3/1
  v_pre/1 -> Product2/2
  Gain6/1 -> Max/1
  Constant/1 -> Max/2
  Pgain Lookup2/1 -> Discrete PID Controller/2
  Discrete PID Controller/1 -> Abs/1
  v_ego/1 -> Gain/1
  Max/1 -> Scope/1, LPF_10rads/1(In1)
  Gain/1 -> Pgain Lookup2/1

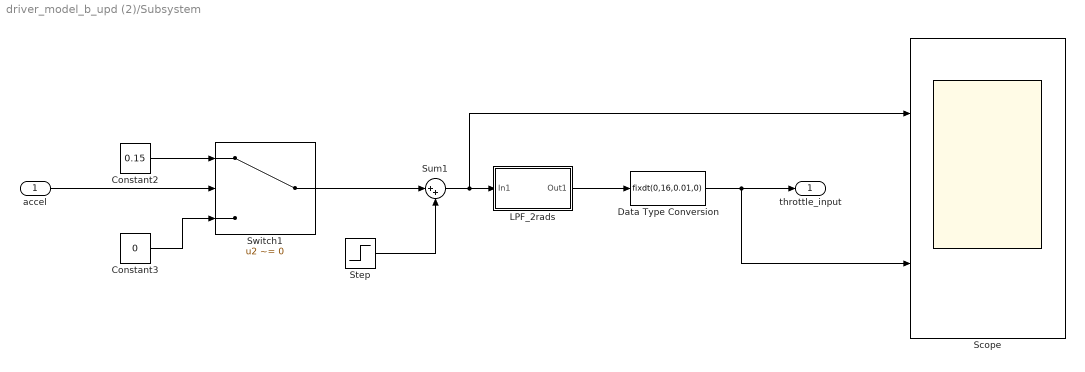
== system driver_model_b_upd (2)/Subsystem ==
  accel : Inport
  Constant2 : Constant  Value=0.15
  Constant3 : Constant  Value=0
  Data Type Conversion : DataTypeConversion  OutDataTypeStr=fixdt(0,16,0.01,0)  SaturateOnIntegerOverflow=off  RndMeth=Floor
  LPF_2rads : Subsystem
  Scope : Scope  NumInputPorts=2
  Step : Step  Time=35  Before=0.2  After=0  SampleTime=0.01
  Sum1 : Sum  Inputs=|++
  Switch1 : Switch  Criteria=u2 ~= 0  SaturateOnIntegerOverflow=off  InputSameDT=off
  throttle_input : Outport
  wires:
  Step/1 -> Sum1/2
  accel/1 -> Switch1/2
  Constant2/1 -> Switch1/1
  Switch1/1 -> Sum1/1
  Constant3/1 -> Switch1/3
  Sum1/1 -> Scope/1, LPF_2rads/1(In1)
  LPF_2rads/1(Out1) -> Data Type Conversion/1
  Data Type Conversion/1 -> Scope/2, throttle_input/1

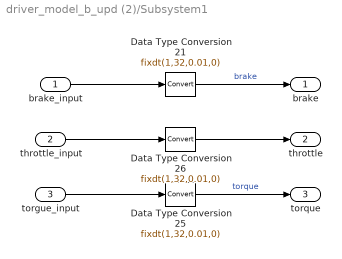
== system driver_model_b_upd (2)/Subsystem1 ==
  brake_input : Inport
  throttle_input : Inport  Port=2
  torgue_input : Inport  Port=3
  Data Type Conversion21 : DataTypeConversion  OutDataTypeStr=fixdt(1,32,0.01,0)  SaturateOnIntegerOverflow=off  RndMeth=Floor
  Data Type Conversion25 : DataTypeConversion  OutDataTypeStr=fixdt(1,32,0.01,0)  SaturateOnIntegerOverflow=off  RndMeth=Floor
  Data Type Conversion26 : DataTypeConversion  OutDataTypeStr=fixdt(1,32,0.01,0)  SaturateOnIntegerOverflow=off  RndMeth=Floor
  brake : Outport
  throttle : Outport  Port=2
  torque : Outport  Port=3
  wires:
  Data Type Conversion21/1 -> brake/1  "brake"
  throttle_input/1 -> Data Type Conversion26/1
  Data Type Conversion25/1 -> torque/1  "torque"
  Data Type Conversion26/1 -> throttle/1
  torgue_input/1 -> Data Type Conversion25/1
  brake_input/1 -> Data Type Conversion21/1

== system driver_model_b_upd (2)/del_v ==
  v_ego : Inport
  v_pre : Inport  Port=2
  Data Type Conversion38 : DataTypeConversion  OutMin=[0]  OutMax=[150]  OutDataTypeStr=fixdt(1,16,2^-6)  RndMeth=Simplest  SaturateOnIntegerOverflow=off
  Data Type Conversion39 : DataTypeConversion  OutMin=[0]  OutMax=[300]  OutDataTypeStr=fixdt(1,16,2^-6)  RndMeth=Nearest  SaturateOnIntegerOverflow=off
  Sum3 : Sum  Inputs=-+  AccumDataTypeStr=fixdt(1,16,0.01,2^-6)  OutDataTypeStr=fixdt(1,16,0.01,2^-6)
  delta_v : Outport
  wires:
  v_ego/1 -> Data Type Conversion38/1
  Data Type Conversion38/1 -> Sum3/1
  Sum3/1 -> delta_v/1  "delta_v"
  Data Type Conversion39/1 -> Sum3/2
  v_pre/1 -> Data Type Conversion39/1

== system driver_model_b_upd (2)/delta_d ==
  In1 : Inport
  In2 : Inport  Port=2
  Sum2 : Sum  Inputs=-+  OutDataTypeStr=fixdt(1,16,2^-6)
  delta_d(m) : Outport
  wires:
  In1/1 -> Sum2/1
  In2/1 -> Sum2/2
  Sum2/1 -> delta_d(m)/1  "delta_d(m)"

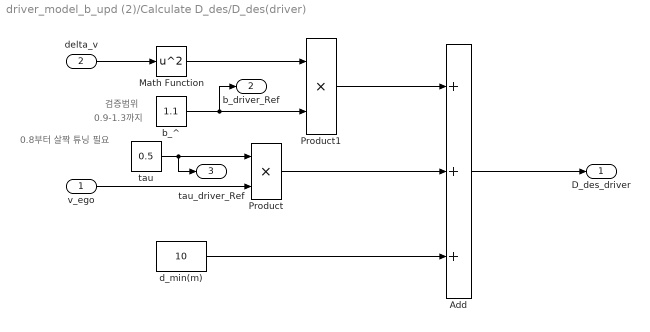
== system driver_model_b_upd (2)/Calculate D_des/D_des(driver) ==
  note: 검증범위
  note: 0.8부터 살짝 튜닝 필요
  note: 0.9-1.3까지
  v_ego : Inport
  delta_v : Inport  Port=2
  Add : Sum  Inputs=+++
  Math Function : Math  Operator=square  SignedPower=on  SaturateOnIntegerOverflow=off
  Product : Product
  Product1 : Product
  b_^ : Constant  Value=1.1
  d_min(m) : Constant  Value=10
  tau : Constant  Value=0.5
  D_des_driver : Outport
  b_driver_Ref : Outport  Port=2
  tau_driver_Ref : Outport  Port=3
  wires:
  Add/1 -> D_des_driver/1
  b_^/1 -> b_driver_Ref/1, Product1/2
  Product/1 -> Add/2
  Math Function/1 -> Product1/1
  delta_v/1 -> Math Function/1
  tau/1 -> tau_driver_Ref/1, Product/1
  v_ego/1 -> Product/2
  Product1/1 -> Add/1
  d_min(m)/1 -> Add/3

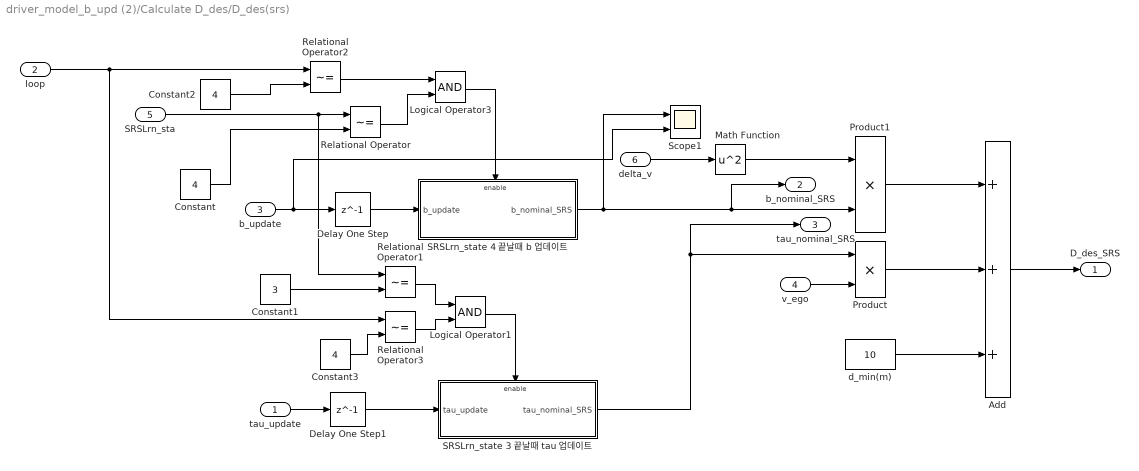
== system driver_model_b_upd (2)/Calculate D_des/D_des(srs) ==
  tau_update : Inport
  loop : Inport  Port=2
  b_update : Inport  Port=3
  v_ego : Inport  Port=4
  SRSLrn_sta : Inport  Port=5
  delta_v : Inport  Port=6
  Add : Sum  Inputs=+++
  Constant : Constant  Value=4
  Constant1 : Constant  Value=3
  Constant2 : Constant  Value=4
  Constant3 : Constant  Value=4
  Delay One Step : Delay  DelayLength=1  InitialCondition=0.5  SampleTime=0.01
  Delay One Step1 : Delay  DelayLength=1  InitialCondition=0.5  SampleTime=0.01
  Logical Operator1 : Logic  AllPortsSameDT=off  OutDataTypeStr=boolean
  Logical Operator3 : Logic  AllPortsSameDT=off  OutDataTypeStr=boolean
  Math Function : Math  Operator=square  SignedPower=on  SaturateOnIntegerOverflow=off
  Product : Product
  Product1 : Product
  Relational Operator{,1..3} (4 alike) : RelationalOperator  Operator=~=  OutDataTypeStr=boolean  InputSameDT=off
  SRSLrn_state 3 끝날때 tau 업데이트 : Subsystem  TreatAsAtomicUnit=on
  SRSLrn_state 4 끝날때 b 업데이트 : Subsystem  TreatAsAtomicUnit=on
  Scope1 : Scope  NumInputPorts=2
  d_min(m) : Constant  Value=10
  D_des_SRS : Outport
  b_nominal_SRS : Outport  Port=2
  tau_nominal_SRS : Outport  Port=3
  wires:
  Product/1 -> Add/2
  Math Function/1 -> Product1/1
  delta_v/1 -> Math Function/1
  d_min(m)/1 -> Add/3
  Product1/1 -> Add/1
  Add/1 -> D_des_SRS/1
  v_ego/1 -> Product/2
  Constant/1 -> Relational Operator/2
  b_update/1 -> Scope1/2, Delay One Step/1
  Delay One Step/1 -> SRSLrn_state 4 끝날때 b 업데이트/1(b_update)
  SRSLrn_state 4 끝날때 b 업데이트/1(b_nominal_SRS) -> Scope1/1, b_nominal_SRS/1, Product1/2
  tau_update/1 -> Delay One Step1/1
  Delay One Step1/1 -> SRSLrn_state 3 끝날때 tau 업데이트/1(tau_update)
  Logical Operator3/1 -> SRSLrn_state 4 끝날때 b 업데이트/Enable
  Constant1/1 -> Relational Operator1/2
  SRSLrn_sta/1 -> Relational Operator1/1, Relational Operator/1
  Relational Operator1/1 -> Logical Operator1/1
  SRSLrn_state 3 끝날때 tau 업데이트/1(tau_nominal_SRS) -> Product/1, tau_nominal_SRS/1
  Constant2/1 -> Relational Operator2/2
  Relational Operator2/1 -> Logical Operator3/1
  Relational Operator/1 -> Logical Operator3/2
  Constant3/1 -> Relational Operator3/2
  loop/1 -> Relational Operator3/1, Relational Operator2/1
  Logical Operator1/1 -> SRSLrn_state 3 끝날때 tau 업데이트/Enable
  Relational Operator3/1 -> Logical Operator1/2

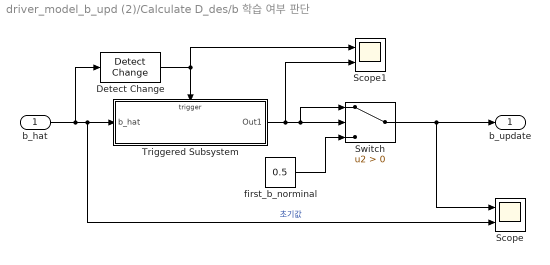
== system driver_model_b_upd (2)/Calculate D_des/b 학습 여부 판단 ==
  b_hat : Inport
  Detect Change : simulink/Logic and Bit Operations/Detect Change  vinit=0  OutDataTypeStr=boolean
  Scope : Scope  NumInputPorts=2
  Scope1 : Scope  NumInputPorts=2
  Switch : Switch  Criteria=u2 > Threshold  SaturateOnIntegerOverflow=off  InputSameDT=off
  Triggered Subsystem : Subsystem  TreatAsAtomicUnit=on
  first_b_norminal : Constant  Value=0.5
  b_update : Outport
  wires:
  first_b_norminal/1 -> Switch/3
  Detect Change/1 -> Triggered Subsystem/Trigger, Scope1/1
  Switch/1 -> Scope/1, b_update/1
  b_hat/1 -> Detect Change/1, Scope/2, Triggered Subsystem/1(b_hat)  "초기값"
  Triggered Subsystem/1(Out1) -> Scope1/2, Switch/1, Switch/2

== system driver_model_b_upd (2)/Calculate D_des/tau 학습 여부 판단 ==
  tau_hat : Inport
  Detect Change : simulink/Logic and Bit Operations/Detect Change  vinit=0  OutDataTypeStr=boolean
  Switch : Switch  Criteria=u2 > Threshold  SaturateOnIntegerOverflow=off  InputSameDT=off
  Triggered Subsystem : Subsystem  TreatAsAtomicUnit=on
  first_tau_norminal : Constant  Value=0.5
  tau_update : Outport
  wires:
  first_tau_norminal/1 -> Switch/3
  Detect Change/1 -> Triggered Subsystem/Trigger
  Switch/1 -> tau_update/1
  Triggered Subsystem/1(Out1) -> Switch/1, Switch/2
  tau_hat/1 -> Detect Change/1, Triggered Subsystem/1(tau_hat)

== system driver_model_b_upd (2)/Driver_brake_input/LPF_10rads ==
  In1 : Inport
  Gain : Gain  Gain=10*0.01
  Subtract : Sum  Inputs=+-
  Subtract1 : Sum
  Unit Delay : UnitDelay  SampleTime=0.01  HasFrameUpgradeWarning=on
  Out1 : Outport
  wires:
  Subtract1/1 -> Out1/1, Unit Delay/1
  Unit Delay/1 -> Subtract/2, Subtract1/2
  Gain/1 -> Subtract1/1
  Subtract/1 -> Gain/1
  In1/1 -> Subtract/1

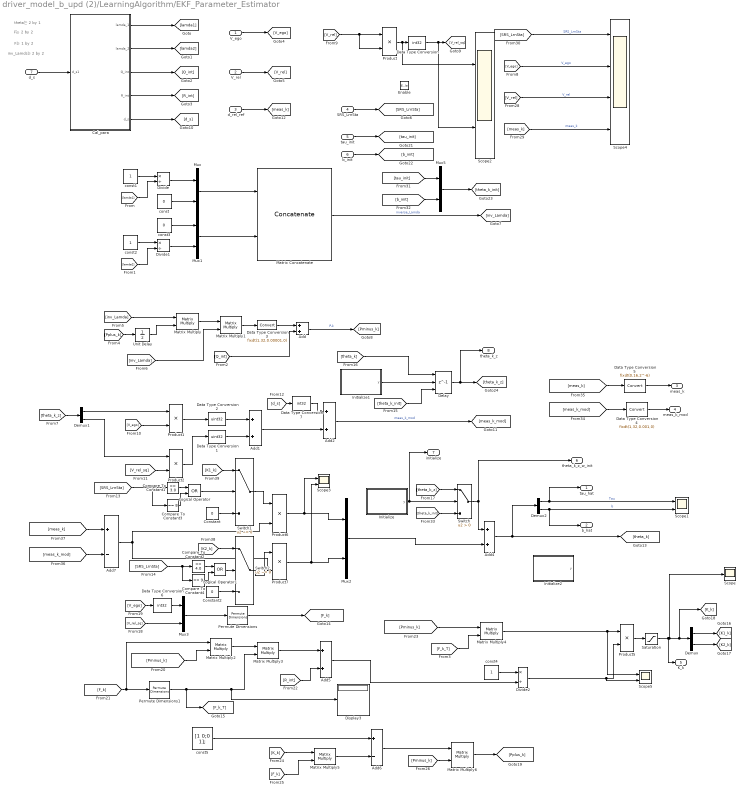
== system driver_model_b_upd (2)/LearningAlgorithm/EKF_Parameter_Estimator ==
  note: inv_Lamda는 2 by 2
  note: theta는 2 by 1
  note: F는 1 by 2
  note: P는 2 by 2
  V_ego : Inport
  V_rel : Inport  Port=2
  d_rel_ref : Inport  Port=3
  SRS_LrnSta : Inport  Port=4
  tau_init : Inport  Port=5
  b_init : Inport  Port=6
  d_s : Inport  Port=7
  Enable : EnablePort  StatesWhenEnabling=reset
  Add{,1..2,4..5} (5 alike) : Sum
  Add6 : Sum  Inputs=+-
  Add7 : Sum  Inputs=+-
  Cal_para : Subsystem
  Compare To Constant1 : simulink/Logic and Bit Operations/Compare To Constant  relop===  const=3.0  OutDataTypeStr=boolean
  Compare To Constant2 : simulink/Logic and Bit Operations/Compare To Constant  relop===  const=4.0  OutDataTypeStr=boolean
  Compare To Constant3 : simulink/Logic and Bit Operations/Compare To Constant  relop===  const=8  OutDataTypeStr=boolean
  Compare To Constant4 : simulink/Logic and Bit Operations/Compare To Constant  relop===  const=9  OutDataTypeStr=boolean
  Constant : Constant  Value=0
  Constant2 : Constant  Value=0
  Data Type Conversion : DataTypeConversion  OutDataTypeStr=int32  SaturateOnIntegerOverflow=off  RndMeth=Floor
  Data Type Conversion1 : DataTypeConversion  OutDataTypeStr=uint32  RndMeth=Floor
  Data Type Conversion2 : DataTypeConversion  OutDataTypeStr=uint32  RndMeth=Floor
  Data Type Conversion3 : DataTypeConversion  OutDataTypeStr=fixdt(1,32,0.00001,0)  RndMeth=Floor
  Data Type Conversion4 : DataTypeConversion  OutDataTypeStr=fixdt(1,32,0.001,0)  SaturateOnIntegerOverflow=off  RndMeth=Floor
  Data Type Conversion5 : DataTypeConversion  OutDataTypeStr=fixdt(0,16,2^-6)  SaturateOnIntegerOverflow=off  RndMeth=Floor
  Data Type Conversion6 : DataTypeConversion  OutDataTypeStr=int32  SaturateOnIntegerOverflow=off  RndMeth=Floor
  Data Type Conversion7 : DataTypeConversion  OutDataTypeStr=int32  SaturateOnIntegerOverflow=off  RndMeth=Floor
  Delay : Delay  DelayLength=1  InitialConditionSource=Input port  ExternalReset=Rising
      settings: InputPortMap=u0,r5,p4
  Demux : Demux  Outputs=2
  Demux1 : Demux  Outputs=2
  Demux2 : Demux  Outputs=2
  Display3 : Display
  Divide : Product  Inputs=*/
  Divide1 : Product  Inputs=*/
  Divide2 : Product  Inputs=*/
  Initialize : Stateflow chart  TreatAsAtomicUnit=on
  Initialize1 : Stateflow chart  TreatAsAtomicUnit=on
  Initialize2 : Stateflow chart  TreatAsAtomicUnit=on
  Logical Operator : Logic  Operator=OR  AllPortsSameDT=off  OutDataTypeStr=boolean
  Logical Operator1 : Logic  Operator=OR  AllPortsSameDT=off  OutDataTypeStr=boolean
  Matrix Concatenate : Concatenate  Mode=Multidimensional array  ConcatenateDimension=2
  Matrix Multiply{,1..6} (7 alike) : Product  Multiplication=Matrix(*)
  Mux{,1..3,5} (5 alike) : Mux  Inputs=2
  Permute Dimensions : PermuteDimensions  Order=[2 1]
  Permute Dimensions1 : PermuteDimensions  Order=[2 1]
  Product{,1..2,5..7} (6 alike) : Product
  Saturation : Saturate  UpperLimit=10000  LowerLimit=0
  Scope : Scope
  Scope{1..3,5} (4 alike) : Scope  NumInputPorts=2
  Scope4 : Scope  NumInputPorts=4
  Switch : Switch  Criteria=u2 > Threshold  SaturateOnIntegerOverflow=off  InputSameDT=off
  Switch1 : Switch  Criteria=u2 ~= 0  SaturateOnIntegerOverflow=off  InputSameDT=off
  Switch2 : Switch  Criteria=u2 ~= 0  SaturateOnIntegerOverflow=off  InputSameDT=off
  Unit Delay : UnitDelay  InitialCondition=[0.001 0;0 0.001]  SampleTime=-1  HasFrameUpgradeWarning=on
  const : Constant  Value=0
  const1 : Constant
  const2 : Constant
  const3 : Constant  Value=0
  const4 : Constant
  const5 : Constant  Value=[1 0;0 1];
  tau_hat : Outport
  b_hat : Outport  Port=2
  meas_k : Outport  Port=3
  meas_k_mod : Outport  Port=4
  K_k : Outport  Port=5
  theta_k_z_w_init : Outport  Port=6
  initialize : Outport  Port=7
  theta_k_z : Outport  Port=8
  wires:
  Data Type Conversion7/1 -> Add2/1
  [d_s] -> Data Type Conversion7/1
  Data Type Conversion3/1 -> Add/1
  d_s/1 -> Cal_para/1(d_s1)
  SRS_LrnSta/1 -> [SRS_LrnSta]
  [Pminus_k] -> Matrix Multiply2/2
  [SRS_LrnSta] -> Compare To Constant3/1, Compare To Constant1/1
  [b_init] -> Mux5/2
  Data Type Conversion6/1 -> Mux3/1
  Matrix Multiply/1 -> Matrix Multiply1/1
  d_rel_ref/1 -> [meas_k]
  Matrix Multiply1/1 -> Data Type Conversion3/1
  [V_ego] -> Product1/2
  Demux1/2 -> Product2/1
  Add1/1 -> Add2/2
  [V_rel_sq] -> Product2/2
  Divide/1 -> Mux/1
  const1/1 -> Divide/1
  Mux1/1 -> Matrix Concatenate/2
  const/1 -> Mux/2
  [lamda1] -> Divide/2
  Demux1/1 -> Product1/1
  Initialize/1(y) -> initialize/1, Switch/2
  Add2/1 -> [meas_k_mod]  "meas_k_mod"
  Divide1/1 -> Mux1/2
  Compare To Constant4/1 -> Logical Operator1/2
  [meas_k] -> Scope4/4  "meas_k"
  Mux2/1 -> Add4/2
  Cal_para/1(lamda_1) -> [lamda1]
  Compare To Constant3/1 -> Logical Operator/2
  Constant2/1 -> Switch2/3
  Demux/2 -> [K2_k]
  Demux2/1 -> tau_hat/1, Scope1/1  "Tau"
  Add5/1 -> Divide2/2
  Compare To Constant1/1 -> Logical Operator/1
  [SRS_LrnSta] -> Compare To Constant4/1, Compare To Constant2/1
  Product/1 -> Scope2/1, Data Type Conversion/1
  Mux/1 -> Matrix Concatenate/1
  Data Type Conversion/1 -> Scope2/2, [V_rel_sq]
  [K2_k] -> Switch2/1
  Demux2/2 -> b_hat/1, Scope1/2  "b"
  [V_rel_sq] -> Mux3/2
  Matrix Concatenate/1 -> [inv_Lamda]  "inverse_Lamda"
  [K1_k] -> Switch1/1
  Logical Operator/1 -> Switch1/2
  const5/1 -> Add6/1
  [lamda2] -> Divide1/2
  [F_k_T] -> Matrix Multiply4/2
  [tau_init] -> Mux5/1
  Permute Dimensions1/1 -> [F_k_T], Display3/1, Matrix Multiply3/2
  [meas_k_mod] -> Add7/2
  [Pminus_k] -> Matrix Multiply4/1
  [R_int] -> Add5/2
  Add7/1 -> Product7/2, Product6/2
  const4/1 -> Divide2/1
  Product6/1 -> Scope3/1, Mux2/1
  V_rel/1 -> [V_rel]
  Switch2/1 -> Product7/1
  Switch1/1 -> Product6/1
  Switch/1 -> theta_k_z_w_init/1, Add4/1
  [meas_k] -> Data Type Conversion5/1
  [inv_Lamda] -> Matrix Multiply/1
  Cal_para/3(Q_int) -> [Q_int]
  Demux/1 -> [K1_k]
  b_init/1 -> [b_init]
  [meas_k] -> Add7/1
  [meas_k_mod] -> Data Type Conversion4/1
  Add/1 -> [Pminus_k]  "P-k"
  Cal_para/4(R_int) -> [R_int]
  [Pplus_k] -> Unit Delay/1
  [Pminus_k] -> Matrix Multiply6/2
  [V_ego] -> Scope4/2  "V_ego"
  [V_rel] -> Scope4/3  "V_rel"
  Mux3/1 -> Permute Dimensions/1
  Permute Dimensions/1 -> [F_k]
  Unit Delay/1 -> Matrix Multiply/2
  Product2/1 -> Data Type Conversion1/1
  Matrix Multiply6/1 -> [Pplus_k]
  [K_k] -> Matrix Multiply5/1
  Divide2/1 -> Scope5/2, Product5/2
  [F_k] -> Matrix Multiply2/1, Permute Dimensions1/1
  Matrix Multiply3/1 -> Add5/1
  [SRS_LrnSta] -> Scope4/1  "SRS_LrnSta"
  Matrix Multiply5/1 -> Add6/2
  Cal_para/2(lamda_2) -> [lamda2]
  [Q_int] -> Add/2
  Matrix Multiply2/1 -> Matrix Multiply3/1
  Product5/1 -> Saturation/1
  [theta_k_z] -> Demux1/1
  [theta_k_z] -> Switch/1
  V_ego/1 -> [V_ego]
  const2/1 -> Divide1/1
  [theta_k_init] -> Switch/3
  Product7/1 -> Scope3/2, Mux2/2
  [F_k] -> Matrix Multiply5/2
  Matrix Multiply4/1 -> Scope5/1, Product5/1
  [V_ego] -> Data Type Conversion6/1
  Saturation/1 -> K_k/1, Scope/1, [K_k], Demux/1
  Constant/1 -> Switch1/3
  Data Type Conversion2/1 -> Add1/1
  Data Type Conversion5/1 -> meas_k/1
  Data Type Conversion1/1 -> Add1/2
  const3/1 -> Mux1/1
  Data Type Conversion4/1 -> meas_k_mod/1
  Logical Operator1/1 -> Switch2/2
  [inv_Lamda] -> Matrix Multiply1/2
  Add6/1 -> Matrix Multiply6/1
  [V_rel] -> Product/2, Product/1
  Add4/1 -> [theta_k], Demux2/1
  Mux5/1 -> [theta_k_init]
  tau_init/1 -> [tau_init]
  Compare To Constant2/1 -> Logical Operator1/1
  Product1/1 -> Data Type Conversion2/1
  Cal_para/5(d_s) -> [d_s]
  Delay/1 -> theta_k_z/1, [theta_k_z]
  [theta_k] -> Delay/1
  Initialize1/1(y) -> Delay/2
  [theta_k_init] -> Delay/3

== system driver_model_b_upd (2)/SRS_regen_input/LPF_10rads ==
  In1 : Inport
  Gain : Gain  Gain=10*0.01
  Subtract : Sum  Inputs=+-
  Subtract1 : Sum
  Unit Delay : UnitDelay  SampleTime=0.01  HasFrameUpgradeWarning=on
  Out1 : Outport
  wires:
  Subtract1/1 -> Out1/1, Unit Delay/1
  Unit Delay/1 -> Subtract/2, Subtract1/2
  Gain/1 -> Subtract1/1
  Subtract/1 -> Gain/1
  In1/1 -> Subtract/1

== system driver_model_b_upd (2)/Subsystem/LPF_2rads ==
  In1 : Inport
  Gain : Gain  Gain=2*0.01
  Subtract : Sum  Inputs=+-
  Subtract1 : Sum
  Unit Delay : UnitDelay  SampleTime=0.01  HasFrameUpgradeWarning=on
  Out1 : Outport
  wires:
  Subtract1/1 -> Out1/1, Unit Delay/1
  Unit Delay/1 -> Subtract/2, Subtract1/2
  Gain/1 -> Subtract1/1
  Subtract/1 -> Gain/1
  In1/1 -> Subtract/1

== system driver_model_b_upd (2)/Calculate D_des/D_des(srs)/SRSLrn_state 3 끝날때 tau 업데이트 ==
  tau_update : Inport
  Enable : EnablePort
  tau_nominal_SRS : Outport
  wires:
  tau_update/1 -> tau_nominal_SRS/1

== system driver_model_b_upd (2)/Calculate D_des/D_des(srs)/SRSLrn_state 4 끝날때 b 업데이트 ==
  b_update : Inport
  Enable : EnablePort
  b_nominal_SRS : Outport
  wires:
  b_update/1 -> b_nominal_SRS/1

== system driver_model_b_upd (2)/Calculate D_des/b 학습 여부 판단/Triggered Subsystem ==
  b_hat : Inport
  Trigger : TriggerPort  TriggerType=falling  VariantControl=(inherit)
  Out1 : Outport
  wires:
  b_hat/1 -> Out1/1

== system driver_model_b_upd (2)/Calculate D_des/tau 학습 여부 판단/Triggered Subsystem ==
  tau_hat : Inport
  Trigger : TriggerPort  TriggerType=falling  VariantControl=(inherit)
  Out1 : Outport
  wires:
  tau_hat/1 -> Out1/1
